simulink model "RUL_system_ML"  (R2021b)
settings: Solver=VariableStepAuto  StartTime=0.0  StopTime=XTest_signal.Time(end)  RelTol=1e-3
settings Model: Creator=tshintai  LastModifiedBy=tshintai

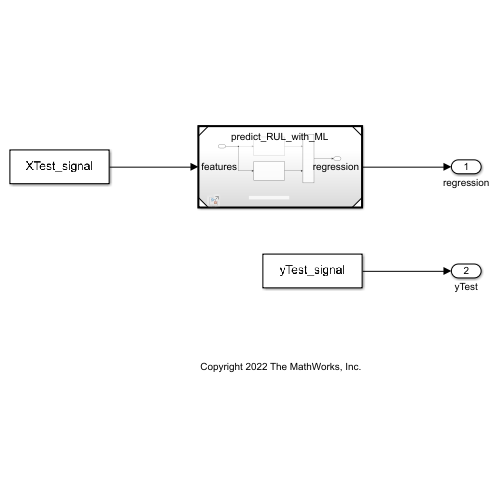
[thumbnail: Simulink's stored preview of the top-level diagram]
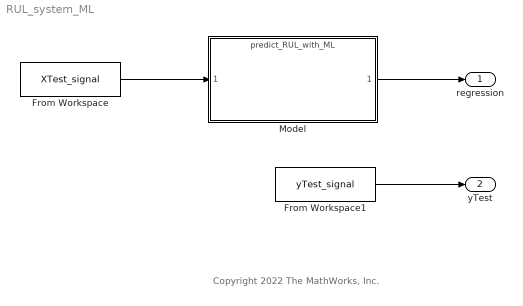
== system RUL_system_ML ==
  note: Copyright 2022 The MathWorks, Inc.
  From Workspace : FromWorkspace  VariableName=XTest_signal  SampleTime=1  Interpolate=off  OutputAfterFinalValue=Holding final value
  From Workspace1 : FromWorkspace  VariableName=yTest_signal  SampleTime=1  Interpolate=off  OutputAfterFinalValue=Holding final value
  Model : ModelReference  ModelNameDialog=predict_RUL_with_ML  SimulationMode=Normal  ModelReferenceVersion=1.14
  regression : Outport
  yTest : Outport  Port=2
  wires:
  From Workspace/1 -> Model/1
  Model/1 -> regression/1
  From Workspace1/1 -> yTest/1
